simulink model "BLDC_motor"  (R2020b)
settings: Solver=VariableStepAuto  StartTime=0.0  StopTime=10.0  RelTol=1e-3
settings Model: Creator=omkar  LastModifiedBy=omkar

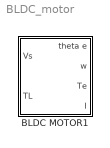
== system BLDC_motor ==
  BLDC MOTOR1 : Subsystem

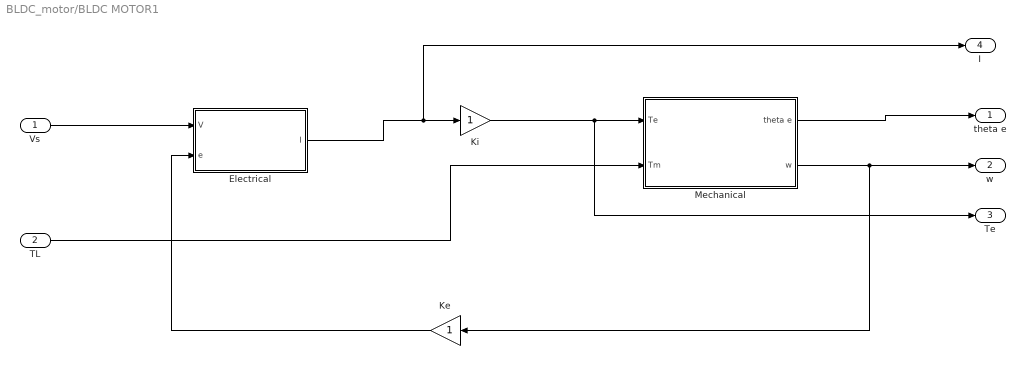
== system BLDC_motor/BLDC MOTOR1 ==
  Vs : Inport
  TL : Inport  Port=2
  Electrical : Subsystem
  Ke : Gain
  Ki : Gain
  Mechanical : Subsystem
  theta e : Outport
  w : Outport  Port=2
  Te : Outport  Port=3
  I : Outport  Port=4
  wires:
  Mechanical/1(theta e) -> theta e/1
  Mechanical/2(w) -> Ke/1, w/1
  Electrical/1(I) -> Ki/1, I/1
  TL/1 -> Mechanical/2(Tm)
  Ki/1 -> Mechanical/1(Te), Te/1
  Vs/1 -> Electrical/1(V)
  Ke/1 -> Electrical/2(e)

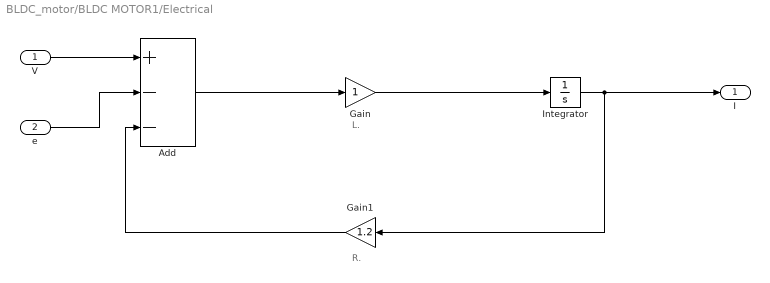
== system BLDC_motor/BLDC MOTOR1/Electrical ==
  note: L.
  note: R.
  V : Inport
  e : Inport  Port=2
  Add : Sum  Inputs=+--
  Gain : Gain
  Gain1 : Gain  Gain=1.2
  Integrator : Integrator
  I : Outport
  wires:
  V/1 -> Add/1
  e/1 -> Add/2
  Gain1/1 -> Add/3
  Gain/1 -> Integrator/1
  Integrator/1 -> Gain1/1, I/1
  Add/1 -> Gain/1

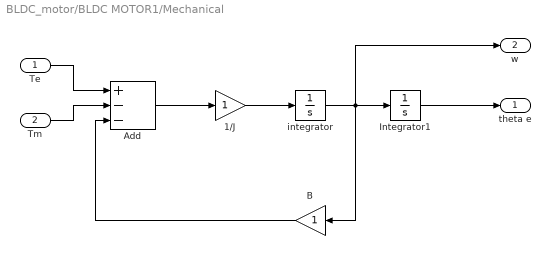
== system BLDC_motor/BLDC MOTOR1/Mechanical ==
  Te : Inport
  Tm : Inport  Port=2
  1/J : Gain
  Add : Sum  Inputs=+--
  B : Gain
  Integrator1 : Integrator
  integrator : Integrator
  theta e : Outport
  w : Outport  Port=2
  wires:
  Add/1 -> 1/J/1
  1/J/1 -> integrator/1
  Tm/1 -> Add/2
  Integrator1/1 -> theta e/1
  B/1 -> Add/3
  integrator/1 -> Integrator1/1, B/1, w/1
  Te/1 -> Add/1
